simulink model "playback_data"  (R2015a)
settings: Solver=FixedStepDiscrete  SolverMode=SingleTasking  StartTime=76  StopTime=110  FixedStep=sample_time  RelTol=1e-3
undefined symbols (not defined in the file): A1_notch_f1, A2_notch_f1, A_kalman_swing_load, A_kalman_transverse, A_kalman_vertical, A_lpf_accelerometer, A_lpf_dtau, A_lpf_fourbar_angles, A_lpf_imu, A_lpf_lateral_angle, B1_lpf_accelerometer, B1_lpf_dtau, B1_lpf_fourbar_angles, B1_lpf_imu, B1_lpf_lateral_angle, B1_notch_f1, B2_lpf_accelerometer, B2_lpf_dtau, B2_lpf_fourbar_angles, B2_lpf_imu, B2_lpf_lateral_angle, B2_notch_f1, B_dx_versus_x0, B_kalman_swing_load, B_kalman_transverse, B_kalman_vertical, backwards_K_sag_of_t, backwards_P_sag_of_t, C_kalman_swing_load, C_kalman_transverse, C_kalman_vertical, com_leg_motor, com_torso, contact_threshold, control_start_time, d_ankle_to_foot, d_vertical_com, desired_com_forward_velocity, desired_com_lateral_velocity, desired_initial_leg_roll_left, desired_initial_leg_roll_right, desired_stance_beta2, desired_standing_torso_pitch, desired_standing_torso_roll, desired_standing_z, desired_torso_pitch, desired_torso_roll, Discrete, enable_bouncing, fcut_contact, fdesignblkfcn, forward_dx_of_dxstar, forward_x_of_dxstar, g, gcbh, HIP_MTR_MAX_CONT_TORQUE, HIP_MTR_MAX_TORQUE, i_leg_motor, i_robot, i_torso ... (+78)
libraries: simulink x65, dsparch4 x18, ctrlSharedLib x14, dspfdesign x4
(part 4 of 13)

== system playback_data/Control1/Filter Velocities ==
  raw dq : Inport
  Demux : Demux  Outputs=3
  Demux1 : Demux  Outputs=3
  Demux2 : Demux  Outputs=2
  Demux3 : Demux  Outputs=2
  Fourbar : Selector  InputPortWidth=13  Indices=[1 2 3 4 5 6 7 8]
  Fourbar Velocity Filter : Scope  NumInputPorts=4
      settings: YMin=-0.55~-0.4~-0.4~-0.6  YMax=0.25~0.7~0.45~0.5  SaveName=ScopeData14  SampleInput=on
  IMU Two Pole Filter : DiscreteTransferFcn  Numerator=[A_lpf_imu 0 0]  Denominator=[1 B1_lpf_imu B2_lpf_imu]  SampleTime=sample_time
  Lateral : Selector  InputPortWidth=13  Indices=[9 10]
  Lateral Angle Two Pole Filter1 : DiscreteTransferFcn  Numerator=[A_lpf_lateral_angle 0 0]  Denominator=[1 B1_lpf_lateral_angle B2_lpf_lateral_angle]  SampleTime=sample_time
  Lateral Angle Two Pole Filter2 : DiscreteTransferFcn  Numerator=[A_lpf_fourbar_angles 0 0]  Denominator=[1 B1_lpf_fourbar_angles B2_lpf_fourbar_angles]  SampleTime=sample_time
  Leg Roll Velocity Filter : Scope  NumInputPorts=2
      settings: YMin=-0.225~-1.5  YMax=0.175~2.25  SaveName=LegRollFilter  SampleInput=on
  Mux : Mux  Inputs=3
  Mux{25..33} (9 alike) : Mux  Inputs=2
  Selector1 : Selector  InputPortWidth=8  Indices=[1 2]
  Selector2 : Selector  InputPortWidth=8  Indices=[3 4]
  Selector3 : Selector  InputPortWidth=8  Indices=[5 6]
  Selector34 : Selector  InputPortWidth=8  Indices=[1 2]
  Selector35 : Selector  InputPortWidth=8  Indices=[3 4]
  Selector36 : Selector  InputPortWidth=8  Indices=[5 6]
  Selector37 : Selector  InputPortWidth=8  Indices=[7 8]
  Selector4 : Selector  InputPortWidth=8  Indices=[7 8]
  Torso Orientation : Selector  InputPortWidth=13  Indices=[11 12 13]
  Torso Orientation Filter : Scope  NumInputPorts=3
      settings: YMin=-0.2~-0.03~-0.15  YMax=0.125~0.0275~0.15  SaveName=ScopeData13  SampleInput=on
  filtered dq : Outport
  wires:
  Lateral Angle Two Pole Filter2/1 -> Selector4/1, Selector3/1, Selector2/1, Selector1/1, Mux/1
  IMU Two Pole Filter/1 -> Demux1/1, Mux/3
  Mux/1 -> filtered dq/1
  raw dq/1 -> Fourbar/1, Torso Orientation/1, Lateral/1
  Lateral/1 -> Demux2/1, Lateral Angle Two Pole Filter1/1
  Torso Orientation/1 -> IMU Two Pole Filter/1, Demux/1
  Lateral Angle Two Pole Filter1/1 -> Demux3/1, Mux/2
  Mux25/1 -> Torso Orientation Filter/1
  Mux27/1 -> Torso Orientation Filter/3
  Mux26/1 -> Torso Orientation Filter/2
  Mux30/1 -> Fourbar Velocity Filter/1
  Mux32/1 -> Fourbar Velocity Filter/3
  Mux31/1 -> Fourbar Velocity Filter/2
  Mux33/1 -> Fourbar Velocity Filter/4
  Selector34/1 -> Mux30/1
  Fourbar/1 -> Selector34/1, Selector35/1, Selector36/1, Selector37/1, Lateral Angle Two Pole Filter2/1
  Selector35/1 -> Mux31/1
  Selector36/1 -> Mux32/1
  Selector37/1 -> Mux33/1
  Mux28/1 -> Leg Roll Velocity Filter/1
  Mux29/1 -> Leg Roll Velocity Filter/2
  Demux/1 -> Mux25/1
  Demux/2 -> Mux26/1
  Demux/3 -> Mux27/1
  Demux1/1 -> Mux25/2
  Demux1/2 -> Mux26/2
  Demux1/3 -> Mux27/2
  Demux2/2 -> Mux29/1
  Demux2/1 -> Mux28/1
  Demux3/1 -> Mux28/2
  Demux3/2 -> Mux29/2
  Selector4/1 -> Mux33/2
  Selector3/1 -> Mux32/2
  Selector2/1 -> Mux31/2
  Selector1/1 -> Mux30/2

== system playback_data/Control/Actuator Control with Torque SEA commands/Compare SEA Signals ==
  Desired : Inport
  Measured : Inport  Port=2
  Demux : Demux
  Demux1 : Demux
  Mux{6..9} (4 alike) : Mux  Inputs=2
  RB : Outport
  RF : Outport  Port=2
  LB : Outport  Port=3
  LF : Outport  Port=4
  wires:
  Demux/3 -> Mux8/1
  Demux/2 -> Mux7/1
  Demux1/1 -> Mux6/2
  Demux/1 -> Mux6/1
  Demux/4 -> Mux9/1
  Demux1/4 -> Mux9/2
  Measured/1 -> Demux1/1
  Demux1/2 -> Mux7/2
  Desired/1 -> Demux/1
  Demux1/3 -> Mux8/2
  Mux6/1 -> RB/1
  Mux7/1 -> RF/1
  Mux9/1 -> LF/1
  Mux8/1 -> LB/1

== system playback_data/Control/Actuator Control with Torque SEA commands/Compare Signals ==
  Measurement : Inport
  Filtered : Inport  Port=2
  Expected : Inport  Port=3
  Demux : Demux
  Demux1 : Demux
  Demux2 : Demux
  Mux{6..9} (4 alike) : Mux  Inputs=3
  RB : Outport
  RF : Outport  Port=2
  LB : Outport  Port=3
  LF : Outport  Port=4
  wires:
  Mux8/1 -> LB/1
  Mux9/1 -> LF/1
  Mux7/1 -> RF/1
  Mux6/1 -> RB/1
  Demux1/3 -> Mux8/2
  Measurement/1 -> Demux/1
  Demux1/2 -> Mux7/2
  Filtered/1 -> Demux1/1
  Demux1/4 -> Mux9/2
  Demux/4 -> Mux9/1
  Demux/1 -> Mux6/1
  Demux1/1 -> Mux6/2
  Demux/2 -> Mux7/1
  Demux/3 -> Mux8/1
  Expected/1 -> Demux2/1
  Demux2/1 -> Mux6/3
  Demux2/2 -> Mux7/3
  Demux2/3 -> Mux8/3
  Demux2/4 -> Mux9/3

== system playback_data/Control/Actuator Control with Torque SEA commands/Compare Torque Derivative Signals ==
  Measured : Inport
  Filtered : Inport  Port=2
  Expected : Inport  Port=3
  Demux : Demux
  Demux1 : Demux
  Demux2 : Demux
  Mux{6..9} (4 alike) : Mux  Inputs=3
  RB : Outport
  RF : Outport  Port=2
  LB : Outport  Port=3
  LF : Outport  Port=4
  wires:
  Demux2/4 -> Mux9/3
  Demux2/3 -> Mux8/3
  Demux2/2 -> Mux7/3
  Demux2/1 -> Mux6/3
  Expected/1 -> Demux2/1
  Demux/3 -> Mux8/1
  Demux/2 -> Mux7/1
  Demux1/1 -> Mux6/2
  Demux/1 -> Mux6/1
  Demux/4 -> Mux9/1
  Demux1/4 -> Mux9/2
  Filtered/1 -> Demux1/1
  Demux1/2 -> Mux7/2
  Measured/1 -> Demux/1
  Demux1/3 -> Mux8/2
  Mux6/1 -> RB/1
  Mux7/1 -> RF/1
  Mux9/1 -> LF/1
  Mux8/1 -> LB/1

== system playback_data/Control/Actuator Control with Torque SEA commands/Compare Velocities ==
  Desired : Inport
  Measured : Inport  Port=2
  Demux : Demux
  Demux1 : Demux
  Mux{6..9} (4 alike) : Mux  Inputs=2
  RB : Outport
  RF : Outport  Port=2
  LB : Outport  Port=3
  LF : Outport  Port=4
  wires:
  Demux1/3 -> Mux8/2
  Desired/1 -> Demux/1
  Demux1/2 -> Mux7/2
  Measured/1 -> Demux1/1
  Demux1/4 -> Mux9/2
  Demux/4 -> Mux9/1
  Demux/1 -> Mux6/1
  Demux1/1 -> Mux6/2
  Demux/2 -> Mux7/1
  Demux/3 -> Mux8/1
  Mux6/1 -> RB/1
  Mux7/1 -> RF/1
  Mux8/1 -> LB/1
  Mux9/1 -> LF/1

== system playback_data/Control/Actuator Control with Torque SEA commands/Contact Velocities ==
  Contact [1/0] x4 : Inport
  Velocities [rad/s] x4 : Inport  Port=2
  Demux : Demux
  Demux1 : Demux
  Mux : Mux
  Velocity on Contact : Subsystem
  Velocity on Contact1 : Subsystem
  Velocity on Contact2 : Subsystem
  Velocity on Contact3 : Subsystem
  Contact Velocities [rad/s] x4 : Outport
  wires:
  Mux/1 -> Contact Velocities [rad/s] x4/1
  Demux/2 -> Velocity on Contact1/Trigger
  Velocity on Contact/1(out) -> Mux/1
  Contact [1/0] x4/1 -> Demux/1
  Velocity on Contact1/1(out) -> Mux/2
  Demux/3 -> Velocity on Contact2/Trigger
  Demux/4 -> Velocity on Contact3/Trigger
  Demux/1 -> Velocity on Contact/Trigger
  Velocity on Contact3/1(out) -> Mux/4
  Velocity on Contact2/1(out) -> Mux/3
  Velocities [rad/s] x4/1 -> Demux1/1
  Demux1/1 -> Velocity on Contact/1(in)
  Demux1/2 -> Velocity on Contact1/1(in)
  Demux1/3 -> Velocity on Contact2/1(in)
  Demux1/4 -> Velocity on Contact3/1(in)

== system playback_data/Control/Actuator Control with Torque SEA commands/Desired Torque Derivative ==
  Signal x4 : Inport
  Reset [1/0] x4 : Inport  Port=2
  Demux : Demux
  Demux1 : Demux
  Gain1 : Gain  Gain=1/sample_time
  Logical Operator : Logic  Operator=NOT  AllPortsSameDT=off  OutDataTypeStr=boolean
  Mux : Mux
  Product : Product
  difference : simulink/Discrete/Difference  ICPrevInput=0.0  InputProcessing=Inherited  OutMin=[]  OutMax=[]  OutDataType=fixdt(1, 16)  OutScaling=2^-10  DoSatur=off
  two_pole_filter{,1..3} (4 alike) : DiscreteTransferFcn  Numerator=[A_lpf_dtau 0 0]  Denominator=[1 B1_lpf_dtau B2_lpf_dtau]  ExternalReset=Rising  SampleTime=sample_time
      settings: InputPortMap=u0,r7
  Derivative x4 : Outport
  wires:
  Demux/1 -> two_pole_filter/1
  difference/1 -> Product/1
  Mux/1 -> Derivative x4/1
  Signal x4/1 -> Gain1/1
  Gain1/1 -> difference/1
  Logical Operator/1 -> Product/2
  Reset [1/0] x4/1 -> Demux1/1, Logical Operator/1
  two_pole_filter/1 -> Mux/1
  Product/1 -> Demux/1
  two_pole_filter1/1 -> Mux/2
  two_pole_filter2/1 -> Mux/3
  two_pole_filter3/1 -> Mux/4
  Demux/2 -> two_pole_filter1/1
  Demux/3 -> two_pole_filter2/1
  Demux/4 -> two_pole_filter3/1
  Demux1/1 -> two_pole_filter/2
  Demux1/2 -> two_pole_filter1/2
  Demux1/3 -> two_pole_filter2/2
  Demux1/4 -> two_pole_filter3/2

== system playback_data/Control/Actuator Control with Torque SEA commands/Expected Forces on Foot ==
  R/L Leg Length [m] x2 : Inport
  R/L Leg Width [m] x2 : Inport  Port=2
  Torques on Load [Nm] x4 : Inport  Port=3
  Divide : Product  Inputs=/*
  Divide1 : Product  Inputs=/*
  Gain3 : Gain  Gain=-1
  Gain6 : Gain  Gain=-1
  Selector2 : Selector  InputPortWidth=4  Indices=[1 3]
  Selector7 : Selector  InputPortWidth=4  Indices=[2 4]
  Sum5 : Sum  Inputs=|-+
  Sum6 : Sum  Inputs=++|
  R/L Orthogonal Force [N] x2 : Outport
  R/L Axial Force [N] x2 : Outport  Port=2
  wires:
  Gain6/1 -> R/L Orthogonal Force [N] x2/1
  Gain3/1 -> R/L Axial Force [N] x2/1
  Sum5/1 -> Divide1/2
  Selector7/1 -> Sum6/2, Sum5/2
  Sum6/1 -> Divide/2
  Selector2/1 -> Sum5/1, Sum6/1
  Divide1/1 -> Gain3/1
  Torques on Load [Nm] x4/1 -> Selector2/1, Selector7/1
  R/L Leg Width [m] x2/1 -> Divide1/1
  R/L Leg Length [m] x2/1 -> Divide/1
  Divide/1 -> Gain6/1

== system playback_data/Control/Actuator Control with Torque SEA commands/Load Torque Kalman Filter ==
  Measured Spring Torque [Nm] x4 : Inport
  Load Position [rad/s] x4 : Inport  Port=2
  Load Velocity [rad/s] x4 : Inport  Port=3
  Reset [1/0] x4 : Inport  Port=4
  Constant{,1..3} (4 alike) : Constant  Value=P0_kalman_swing_load
  Demux2 : Demux
  Difference{,1..3} (4 alike) : simulink/Discrete/Difference  ICPrevInput=0.0  InputProcessing=Inherited  OutMin=[]  OutMax=[]  OutDataType=fixdt(1, 16)  OutScaling=2^-10  DoSatur=off
  Gain{1..4} (4 alike) : Gain  Gain=1/mean(j_segments)
  Gain5 : Gain  Gain=mean(j_segments)
  MATLAB Function : MATLAB Function  TreatAsAtomicUnit=on
  Mux : Mux
  Mux{1,3,5,7} (4 alike) : Mux  Inputs=2
  Mux{2,4,6,8} (4 alike) : Mux  Inputs=3
  Selector : Selector  InputPortWidth=4  Indices=[1]
  Selector{1..3,12} (4 alike) : Selector  InputPortWidth=3  Indices=[3]
  Selector10 : Selector  InputPortWidth=4  Indices=[2]
  Selector11 : Selector  InputPortWidth=4  Indices=[3]
  Selector13 : Selector  InputPortWidth=4  Indices=[3]
  Selector14 : Selector  InputPortWidth=4  Indices=[4]
  Selector15 : Selector  InputPortWidth=4  Indices=[4]
  Selector4 : Selector  InputPortWidth=4  Indices=[1]
  Selector5 : Selector  InputPortWidth=4  Indices=[1]
  Selector6 : Selector  InputPortWidth=4  Indices=[2]
  Selector7 : Selector  InputPortWidth=4  Indices=[3]
  Selector8 : Selector  InputPortWidth=4  Indices=[4]
  Selector9 : Selector  InputPortWidth=4  Indices=[2]
  Swing Load Kalman Filter{,1..3} (4 alike) : ctrlSharedLib/Kalman Filter  TimeDomain=Discrete-Time  UseCurrentEstimator=on  ModelSource=Individual A, B, C, D matrices  ModelSourceVariable=A_kf  A=A_kalman_swing_load  B=B_kalman_swing_load  C=C_kalman_swing_load  D=0  NumberOfStates=2  NumberOfInputs=1  NumberOfOutputs=2  InitialEstimateSource=Input port  X0=initial_dx_estimate  P0=P0_kalman_transverse  UseK=off  UseGH=on  NumberOfProcessNoiseInputs=1  G=G_kalman_swing_load  TimeInvariantG=on  H=0  TimeInvariantH=on  Q=Q_kalman_SEA_torque_difference  TimeInvariantQ=on  R=1  TimeInvariantR=off  N=0  TimeInvariantN=on  AddInputPort=on  AddEnablePort=off  ExternalReset=Rising  OutputEstimatedY=off  OutputP=off  Ts=sample_time
  Load Torques [Nm] x4 : Outport
  wires:
  Mux6/1 -> Swing Load Kalman Filter/3
  Mux5/1 -> Swing Load Kalman Filter/2
  Difference/1 -> Swing Load Kalman Filter/1
  Demux2/1 -> Gain3/1, Mux5/2, Difference/1
  Swing Load Kalman Filter/1 -> Selector12/1
  Selector12/1 -> Mux/1
  Mux2/1 -> Swing Load Kalman Filter1/3
  Mux1/1 -> Swing Load Kalman Filter1/2
  Difference1/1 -> Swing Load Kalman Filter1/1
  Demux2/2 -> Gain1/1, Mux1/2, Difference1/1
  Gain1/1 -> Mux2/3
  Mux4/1 -> Swing Load Kalman Filter2/3
  Mux3/1 -> Swing Load Kalman Filter2/2
  Difference2/1 -> Swing Load Kalman Filter2/1
  Demux2/3 -> Difference2/1, Mux3/2, Gain2/1
  Gain2/1 -> Mux4/3
  Mux8/1 -> Swing Load Kalman Filter3/3
  Mux7/1 -> Swing Load Kalman Filter3/2
  Difference3/1 -> Swing Load Kalman Filter3/1
  Demux2/4 -> Difference3/1, Mux7/2, Gain4/1
  Gain4/1 -> Mux8/3
  Swing Load Kalman Filter1/1 -> Selector1/1
  Swing Load Kalman Filter3/1 -> Selector3/1
  Swing Load Kalman Filter2/1 -> Selector2/1
  Mux/1 -> Gain5/1
  Selector1/1 -> Mux/2
  Selector2/1 -> Mux/3
  Selector3/1 -> Mux/4
  Reset [1/0] x4/1 -> [Reset]
  Load Velocity [rad/s] x4/1 -> [LoadVelocities]
  Measured Spring Torque [Nm] x4/1 -> MATLAB Function/1(spring_torques), Demux2/1
  Gain5/1 -> Load Torques [Nm] x4/1
  Gain3/1 -> Mux6/3
  Load Position [rad/s] x4/1 -> [LoadPositions]
  [LoadPositions] -> Selector/1
  [LoadVelocities] -> Selector4/1
  Selector/1 -> Mux6/1, Mux5/1
  Selector4/1 -> Mux6/2
  [Reset] -> Selector5/1
  Selector5/1 -> Swing Load Kalman Filter/5
  [Reset] -> Selector6/1
  Selector6/1 -> Swing Load Kalman Filter1/5
  [Reset] -> Selector7/1
  Selector7/1 -> Swing Load Kalman Filter2/5
  [Reset] -> Selector8/1
  Selector8/1 -> Swing Load Kalman Filter3/5
  [LoadVelocities] -> Selector9/1
  [LoadPositions] -> Selector10/1
  [LoadVelocities] -> Selector11/1
  [LoadPositions] -> Selector13/1
  [LoadVelocities] -> Selector14/1
  [LoadPositions] -> Selector15/1
  Selector15/1 -> Mux8/1, Mux7/1
  Selector13/1 -> Mux4/1, Mux3/1
  Selector11/1 -> Mux4/2
  Selector14/1 -> Mux8/2
  Selector9/1 -> Mux2/2
  Selector10/1 -> Mux2/1, Mux1/1
  Constant/1 -> Swing Load Kalman Filter1/4
  MATLAB Function/1(R1) -> [R1]
  MATLAB Function/2(R2) -> [R2]
  MATLAB Function/3(R3) -> [R3]
  MATLAB Function/4(R4) -> [R4]
  [R2] -> Swing Load Kalman Filter1/6
  [R1] -> Swing Load Kalman Filter/6
  Constant1/1 -> Swing Load Kalman Filter/4
  [R3] -> Swing Load Kalman Filter2/6
  Constant2/1 -> Swing Load Kalman Filter2/4
  Constant3/1 -> Swing Load Kalman Filter3/4
  [R4] -> Swing Load Kalman Filter3/6

== system playback_data/Control/Actuator Control with Torque SEA commands/Lowpass Filter ==
  In : Inport
  Generated Filter Block : dsparch4/Biquad Filter  Tag=BlockMethodSubSystem  IIRFiltStruct=Direct form II  CoeffSource=Specify via dialog  BiQuadCoeffs=[1.0054190789171848 -2 1.0054190789171853 1 -1.9557970115108714 0.95685429506963915]  a0Flag=Warning  IC=0  ICnum=0  ICden=0  denAccumFracLength=30  denProdOutputFracLength=30  secondMemoryFracLength=15  roundingMode=Floor  overflowMode=off  ScaleValues=[0.0010519560093213882;92.733879468734756]  optimizeScaleValues=off  ScaleValueMode=Specify via input port (g)  scaleValueFracLength=14  FilterSource=Specify via dialog  FilterObject=Hm_biquad
  Out : Outport
  wires:
  Generated Filter Block/1 -> Out/1
  In/1 -> Generated Filter Block/1

== system playback_data/Control/Actuator Control with Torque SEA commands/Lowpass Filter1 ==
  In : Inport
  Generated Filter Block : dsparch4/Biquad Filter  Tag=BlockMethodSubSystem  IIRFiltStruct=Direct form II  CoeffSource=Specify via dialog  BiQuadCoeffs=[1.0054190789171848 -2 1.0054190789171853 1 -1.9557970115108714 0.95685429506963915]  a0Flag=Warning  IC=0  ICnum=0  ICden=0  denAccumFracLength=30  denProdOutputFracLength=30  secondMemoryFracLength=15  roundingMode=Floor  overflowMode=off  ScaleValues=[0.0010519560093213882;92.733879468734756]  optimizeScaleValues=off  ScaleValueMode=Specify via input port (g)  scaleValueFracLength=14  FilterSource=Specify via dialog  FilterObject=Hm_biquad
  Out : Outport
  wires:
  In/1 -> Generated Filter Block/1
  Generated Filter Block/1 -> Out/1

== system playback_data/Control/Actuator Control with Torque SEA commands/Lowpass Filter2 ==
  In : Inport
  Generated Filter Block : dsparch4/Biquad Filter  Tag=BlockMethodSubSystem  IIRFiltStruct=Direct form II  CoeffSource=Specify via dialog  BiQuadCoeffs=[0.42638734887522584 0.71004939850960869 0.42638734887522595 1 0.054295561672899631 0.19751119790393634]  a0Flag=Warning  IC=0  ICnum=0  ICden=0  denAccumFracLength=30  denProdOutputFracLength=30  secondMemoryFracLength=15  roundingMode=Floor  overflowMode=off  ScaleValues=[0.80099018345858064;1]  optimizeScaleValues=off  ScaleValueMode=Specify via input port (g)  scaleValueFracLength=14  FilterSource=Specify via dialog  FilterObject=Hm_biquad
  Out : Outport
  wires:
  In/1 -> Generated Filter Block/1
  Generated Filter Block/1 -> Out/1

== system playback_data/Control/Actuator Control with Torque SEA commands/Lowpass Filter5 ==
  In : Inport
  Generated Filter Block : dsparch4/Biquad Filter  Tag=BlockMethodSubSystem  IIRFiltStruct=Direct form II  CoeffSource=Specify via dialog  BiQuadCoeffs=[1.0054190789171848 -2 1.0054190789171853 1 -1.9557970115108714 0.95685429506963915]  a0Flag=Warning  IC=0  ICnum=0  ICden=0  denAccumFracLength=30  denProdOutputFracLength=30  secondMemoryFracLength=15  roundingMode=Floor  overflowMode=off  ScaleValues=[0.0010519560093213882;92.733879468734756]  optimizeScaleValues=off  ScaleValueMode=Specify via input port (g)  scaleValueFracLength=14  FilterSource=Specify via dialog  FilterObject=Hm_biquad
  Out : Outport
  wires:
  In/1 -> Generated Filter Block/1
  Generated Filter Block/1 -> Out/1

== system playback_data/Control/Actuator Control with Torque SEA commands/Lowpass Filter6 ==
  In : Inport
  Generated Filter Block : dsparch4/Biquad Filter  Tag=BlockMethodSubSystem  IIRFiltStruct=Direct form II  CoeffSource=Specify via dialog  BiQuadCoeffs=[1.0054190789171848 -2 1.0054190789171853 1 -1.9557970115108714 0.95685429506963915]  a0Flag=Warning  IC=0  ICnum=0  ICden=0  denAccumFracLength=30  denProdOutputFracLength=30  secondMemoryFracLength=15  roundingMode=Floor  overflowMode=off  ScaleValues=[0.0010519560093213882;92.733879468734756]  optimizeScaleValues=off  ScaleValueMode=Specify via input port (g)  scaleValueFracLength=14  FilterSource=Specify via dialog  FilterObject=Hm_biquad
  Out : Outport
  wires:
  Generated Filter Block/1 -> Out/1
  In/1 -> Generated Filter Block/1

== system playback_data/Control/Actuator Control with Torque SEA commands/Measured Forces on Foot ==
  R/L Leg Length [m] x2 : Inport
  R/L Leg Width [m] x2 : Inport  Port=2
  Torques on Load [Nm] x4 : Inport  Port=3
  Divide : Product  Inputs=/*
  Divide1 : Product  Inputs=/*
  Gain3 : Gain  Gain=-1
  Gain6 : Gain  Gain=-1
  Selector2 : Selector  InputPortWidth=4  Indices=[1 3]
  Selector7 : Selector  InputPortWidth=4  Indices=[2 4]
  Sum5 : Sum  Inputs=|-+
  Sum6 : Sum  Inputs=++|
  R/L Orthogonal Force [N] x2 : Outport
  R/L Axial Force [N] x2 : Outport  Port=2
  wires:
  Divide/1 -> Gain6/1
  R/L Leg Length [m] x2/1 -> Divide/1
  R/L Leg Width [m] x2/1 -> Divide1/1
  Torques on Load [Nm] x4/1 -> Selector7/1, Selector2/1
  Divide1/1 -> Gain3/1
  Selector2/1 -> Sum6/1, Sum5/1
  Sum6/1 -> Divide/2
  Selector7/1 -> Sum5/2, Sum6/2
  Sum5/1 -> Divide1/2
  Gain3/1 -> R/L Axial Force [N] x2/1
  Gain6/1 -> R/L Orthogonal Force [N] x2/1

== system playback_data/Control/Actuator Control with Torque SEA commands/SEA Controller (Torque) ==
  phi_load [rad] x4 : Inport
  phi_gear [rad] x4 : Inport  Port=2
  dphi_load [rad/s] x4 : Inport  Port=3
  dphi_gear [rad/s] x4 : Inport  Port=4
  tau_des sagittal [Nm] x4 : Inport  Port=5
  dtau_des sagittal [Nm] x4 : Inport  Port=6
  Abs : Abs
  Antiresonance Compensation : Subsystem
  Friction Compensation : Subsystem
  Loaded Unloaded Switch : Subsystem
  P gain ramp : Lookup_n-D  NumberOfTableDimensions=1  BreakpointsForDimension1=[0,65,350,700]  Table=0.60*[0.3, 0.3, 6.0, 6.0]  InternalRulePriority=Speed  RndMeth=Simplest  InputSameDT=on
  Product : Product  SampleTime=sample_time  RndMeth=Zero
  Product2 : Product  RndMeth=Zero
  Spring Stiffness : Gain  Gain=k_sea_low
  Spring Stiffness 1 : Gain  Gain=k_sea_low
  Sum1 : Sum  Inputs=-+|
  Sum10 : Sum  Inputs=|++
  Sum2 : Sum  Inputs=|+-
  Sum3 : Sum  Inputs=++|
  Sum5 : Sum  Inputs=|+-
  Sum6 : Sum  Inputs=-+|
  Sum7 : Sum  Inputs=+|+
  Torque Limiter (outside) 1 : Saturate  UpperLimit=max_sagittal_loaded_torque  LowerLimit=-max_sagittal_loaded_torque
      settings: AttributesFormatString=Hi: %<UpperLimit>\nLo: %<LowerLimit>
  Torque Limiter (outside) 3 : Saturate  UpperLimit=max_sagittal_unloaded_torque  LowerLimit=-max_sagittal_unloaded_torque
      settings: AttributesFormatString=Hi: %<UpperLimit>\nLo: %<LowerLimit>
  Torque Threshold : simulink/Logic and Bit Operations/Compare To Constant  relop=>=  const=loaded_unloaded_torque_threshold  OutDataTypeStr=boolean
  critical damping : Subsystem
  tau_cmd sagittal [Nm] x4 : Outport
  tau_measured [Nm] x4 : Outport  Port=2
  wires:
  Product2/1 -> Sum7/2
  Sum2/1 -> Product2/2
  Sum5/1 -> Product/2
  dphi_gear [rad/s] x4/1 -> Friction Compensation/1(Motor Velocity [rad/s]), Sum6/2
  dphi_load [rad/s] x4/1 -> Sum6/1
  Spring Stiffness 1/1 -> Sum2/2
  Sum6/1 -> Spring Stiffness 1/1
  dtau_des sagittal [Nm] x4/1 -> Sum2/1
  tau_des sagittal [Nm] x4/1 -> Sum5/1
  phi_gear [rad] x4/1 -> Sum1/2
  phi_load [rad] x4/1 -> Sum1/1
  Sum1/1 -> Spring Stiffness/1
  Spring Stiffness/1 -> Sum3/1, Sum5/2, Abs/1, tau_measured [Nm] x4/1
  Sum10/1 -> Antiresonance Compensation/1(Torque), Torque Limiter (outside) 1/1
  P gain ramp/1 -> critical damping/1(p gain), Product/1
  Product/1 -> Sum7/1
  Sum7/1 -> Sum3/2
  Torque Limiter (outside) 1/1 -> Loaded Unloaded Switch/1(Loaded Signal)
  Torque Limiter (outside) 3/1 -> Loaded Unloaded Switch/2(Unloaded Signal)
  Antiresonance Compensation/1(Filtered Torque) -> Torque Limiter (outside) 3/1
  Friction Compensation/1(Friction Compensation [Nm]) -> Sum10/2
  Loaded Unloaded Switch/1(Signal) -> tau_cmd sagittal [Nm] x4/1
  Torque Threshold/1 -> Loaded Unloaded Switch/3(Loaded/Unloaded [1/0] x4)
  Abs/1 -> P gain ramp/1, Torque Threshold/1
  Sum3/1 -> Sum10/1
  critical damping/1(d gain) -> Product2/1

== system playback_data/Control/Actuator Control with Torque SEA commands/SEA Controller (Velocity) ==
  phi_load [rad] x4 : Inport
  phi_gear [rad] x4 : Inport  Port=2
  dphi_load [rad/s] x4 : Inport  Port=3
  tau_des sagittal [Nm] x4 : Inport  Port=4
  dtau_des sagittal [Nm] x4 : Inport  Port=5
  Reset SEA Control [1/0] x4 : Inport  Port=6
  Stance (1) or Swing (0) x4 : Inport  Port=7
  Demux : Demux
  Demux1 : Demux
  Demux2 : Demux
  Feedback : Scope  NumInputPorts=4
      settings: YMin=-4~-0.9~-5~-5  YMax=4.5~1~5~5  SaveName=ScopeData7  SampleInput=on
  Feedforward : Scope  NumInputPorts=4
      settings: YMin=-4~-0.9~-5~-5  YMax=4.5~1~5~5  SaveName=ScopeData4  SampleInput=on
  Gain3 : Gain  Gain=1./k_sea_low
  Integrator : Subsystem
  Kp : Constant  Value=0.016
  Lowpass Filter (Stance) : Subsystem  DialogController=fdesignblkfcn  InitFcn=fdesignblkfcn(gcbh, {'InitFcn'});  mask(Lowpass Filter){}
      mask help: Design a lowpass filter
      settings: CopyFcn=fdesignblkfcn(gcbh, {'CopyFcn'});
      mask Help: helpview(mapfilelocation('dsp'), 'dsplowpassfilter');
      mask Display: disp('Lowpass')
  Lowpass Filter (Swing) : Subsystem  DialogController=fdesignblkfcn  InitFcn=fdesignblkfcn(gcbh, {'InitFcn'});  mask(Lowpass Filter){}
      mask help: Design a lowpass filter
      settings: CopyFcn=fdesignblkfcn(gcbh, {'CopyFcn'});
      mask Help: helpview(mapfilelocation('dsp'), 'dsplowpassfilter');
      mask Display: disp('Lowpass')
  Nonlinear Spring Force : MATLAB Function  TreatAsAtomicUnit=on
  Product : Product
  Stance Swing : Scope  NumInputPorts=4
      settings: YMin=-4~-0.9~-5~-5  YMax=4.5~1~5~5  SaveName=ScopeData5  SampleInput=on
  Stance or Swing : Subsystem
  Stance or Swing1 : Subsystem
  Stance or Swing2 : Subsystem
  Sum1 : Sum  Inputs=-+|
  Sum10 : Sum  Inputs=++|
  Sum4 : Sum  Inputs=|++
  Sum5 : Sum  Inputs=|+-
  Sum6 : Sum  Inputs=|++
  Ti : Gain  Gain=1/0.150
  Torque Limiter (stance) : Saturate  UpperLimit=700  LowerLimit=-700
      settings: AttributesFormatString=Hi: %<UpperLimit>\nLo: %<LowerLimit>
  Torque Limiter (swing) : Saturate  UpperLimit=80  LowerLimit=-80
      settings: AttributesFormatString=Hi: %<UpperLimit>\nLo: %<LowerLimit>
  Velocity Notch Filter (Swing) : dspfdesign/Notch-Peak Filter  Specification=Quality factor and center frequency  Bandwidth=27  QualityFactor=2.5  CenterFrequency=27  BandwidthCoefficient=0.72654  CenterFrequencyCoefficient=0  Output=Notch  InheritSampleRate=off  SampleRate=update_freq  SimulateUsing=Code generation
  Velocity Command [rad/s] x4 : Outport  PortDimensions=4
  tau_measured [Nm] x4 : Outport  Port=2
  wires:
  Sum1/1 -> Nonlinear Spring Force/1(deflections)
  Nonlinear Spring Force/1(tau_sea) -> tau_measured [Nm] x4/1, Sum5/2
  Product/1 -> Ti/1, Sum10/1
  Sum6/1 -> Stance or Swing1/2(Signal True x4), Velocity Notch Filter (Swing)/1
  Gain3/1 -> Sum4/1
  dtau_des sagittal [Nm] x4/1 -> Gain3/1
  Reset SEA Control [1/0] x4/1 -> Integrator/2(Reset [1/0])
  Sum5/1 -> Product/1
  Integrator/1(Integrated) -> Sum10/2
  Ti/1 -> Integrator/1(Signal)
  dphi_load [rad/s] x4/1 -> Sum4/2
  Sum4/1 -> Lowpass Filter (Stance)/1(In), Lowpass Filter (Swing)/1(In)
  Lowpass Filter (Stance)/1(Out) -> Stance or Swing2/2(Signal True x4), Demux1/1
  Kp/1 -> Product/2
  Stance or Swing/1(Selected x4) -> Sum5/1
  Torque Limiter (swing)/1 -> Stance or Swing/3(Signal False x4)
  Torque Limiter (stance)/1 -> Stance or Swing/2(Signal True x4)
  Stance or Swing1/1(Selected x4) -> Velocity Command [rad/s] x4/1
  Velocity Notch Filter (Swing)/1 -> Stance or Swing1/3(Signal False x4)
  Demux/4 -> Feedback/4
  Demux/3 -> Feedback/3
  Demux/2 -> Feedback/2
  Demux/1 -> Feedback/1
  Demux1/1 -> Feedforward/1
  Demux1/2 -> Feedforward/2
  Demux1/3 -> Feedforward/3
  Demux1/4 -> Feedforward/4
  tau_des sagittal [Nm] x4/1 -> Torque Limiter (stance)/1, Torque Limiter (swing)/1
  phi_gear [rad] x4/1 -> Sum1/2
  phi_load [rad] x4/1 -> Sum1/1
  Stance (1) or Swing (0) x4/1 -> Demux2/1, Stance or Swing2/1(True/False x4), Stance or Swing1/1(True/False x4), Stance or Swing/1(True/False x4)
  Demux2/3 -> Stance Swing/3
  Demux2/2 -> Stance Swing/2
  Demux2/1 -> Stance Swing/1
  Demux2/4 -> Stance Swing/4
  Sum10/1 -> Demux/1, Sum6/1
  Lowpass Filter (Swing)/1(Out) -> Stance or Swing2/3(Signal False x4)
  Stance or Swing2/1(Selected x4) -> Sum6/2

== system playback_data/Control/Actuator Control with Torque SEA commands/Stance or Swing1 ==
  True/False x4 : Inport
  Signal True x4 : Inport  Port=2
  Signal False x4 : Inport  Port=3
  Demux : Demux
  Demux1 : Demux
  Demux2 : Demux
  Mux : Mux
  Switch{,1..3} (4 alike) : Switch  Criteria=u2 ~= 0
  Selected x4 : Outport
  wires:
  Switch3/1 -> Mux/4
  Switch2/1 -> Mux/3
  Switch1/1 -> Mux/2
  Switch/1 -> Mux/1
  Demux1/4 -> Switch3/2
  Demux1/3 -> Switch2/2
  Demux1/2 -> Switch1/2
  Demux1/1 -> Switch/2
  Demux2/4 -> Switch3/3
  Demux2/3 -> Switch2/3
  Demux2/2 -> Switch1/3
  Demux2/1 -> Switch/3
  Demux/4 -> Switch3/1
  Demux/3 -> Switch2/1
  Demux/2 -> Switch1/1
  Demux/1 -> Switch/1
  Signal False x4/1 -> Demux2/1
  Signal True x4/1 -> Demux/1
  True/False x4/1 -> Demux1/1
  Mux/1 -> Selected x4/1

== system playback_data/Control/Actuator Control with Torque SEA commands/Timers ==
  Start [1/0] x4 : Inport
  Time [s] : Inport  Port=2
  Demux : Demux
  Mux : Mux
  Sum{8..11} (4 alike) : Sum  Inputs=|-+
  Time on Contact : Subsystem
  Time on Contact1 : Subsystem
  Time on Contact2 : Subsystem
  Time on Contact3 : Subsystem
  Timer [s] x4 : Outport
  wires:
  Sum10/1 -> Mux/3
  Sum11/1 -> Mux/4
  Demux/1 -> Time on Contact/Trigger
  Demux/4 -> Time on Contact3/Trigger
  Demux/3 -> Time on Contact2/Trigger
  Time on Contact3/1(out) -> Sum11/1
  Sum9/1 -> Mux/2
  Start [1/0] x4/1 -> Demux/1
  Sum8/1 -> Mux/1
  Time on Contact1/1(out) -> Sum9/1
  Demux/2 -> Time on Contact1/Trigger
  Time [s]/1 -> Time on Contact3/1(in), Time on Contact2/1(in), Time on Contact1/1(in), Time on Contact/1(in), Sum8/2, Sum9/2, Sum11/2, Sum10/2
  Mux/1 -> Timer [s] x4/1
  Time on Contact2/1(out) -> Sum10/1
  Time on Contact/1(out) -> Sum8/1

== system playback_data/Control/Behavior Control/At Least One Stance Detected ==
  Enable : EnablePort  StatesWhenEnabling=reset
  Constant : Constant
  Stance? : Outport  InitialOutput=[0]
  wires:
  Constant/1 -> Stance?/1

== system playback_data/Control/Behavior Control/Compute Forces1 ==
  XYZ Acceleration : Inport
  Constant5 : Constant  Value=g
  Demux : Demux  Outputs=3
  Gain4 : Gain  Gain=m_total_real
  Mux : Mux  Inputs=3
  Sum8 : Sum  Inputs=|++
  XYZ Force : Outport
  wires:
  Demux/1 -> Mux/1
  Demux/2 -> Mux/2
  Demux/3 -> Sum8/1
  Sum8/1 -> Mux/3
  Mux/1 -> Gain4/1
  Gain4/1 -> XYZ Force/1
  XYZ Acceleration/1 -> Demux/1
  Constant5/1 -> Sum8/2

== system playback_data/Control/Behavior Control/Contact State Machine ==
  Contact Factor [body weight] : Inport
  "[Z dZ] [m m/s]" : Inport  Port=2
  ddZ [m/s^2] : Inport  Port=3
  Contact Factor ddz : Scope
      settings: YMin=-8  YMax=11  SaveName=ScopeData47  SampleInput=on
  Contact State : Scope
      settings: YMin=-0.007  YMax=0.0005  SaveName=ScopeData46  SampleInput=on
  Detect Fall Nonpositive : simulink/Logic and Bit Operations/Detect Fall Nonpositive  vinit=1  InputProcessing=Inherited  OutDataTypeStr=boolean
  Mux : Mux  Inputs=2
  Mux25 : Mux  Inputs=5
  Selector : Selector  InputPortWidth=2  Indices=[2]
  State Machine : State Transition Table  TreatAsAtomicUnit=on
  Unit Delay5 : UnitDelay  SampleTime=-1
  Unit Delay6 : UnitDelay  SampleTime=sample_time
  Unit Delay7 : UnitDelay  InitialCondition=1  SampleTime=sample_time
  flight [1/0] : Outport
  Exiting Stance [1/0] : Outport  Port=2
  wires:
  Detect Fall Nonpositive/1 -> Exiting Stance [1/0]/1
  Unit Delay7/1 -> flight [1/0]/1
  Unit Delay6/1 -> Detect Fall Nonpositive/1
  State Machine/4(" Takeoff") -> Unit Delay6/1, Mux25/4
  Selector/1 -> State Machine/1(z_velocity), Unit Delay5/1
  Contact Factor [body weight]/1 -> Mux/1, State Machine/3(vertical_grf)
  Unit Delay5/1 -> State Machine/2(previous_z_velocity)
  State Machine/5(" Flight") -> Mux25/5, Unit Delay7/1
  Mux25/1 -> Contact State/1
  State Machine/3(" Unloading") -> Mux25/3
  State Machine/2(" LockedContact") -> Mux25/2
  State Machine/1(" TouchDown") -> Mux25/1
  "[Z dZ] [m m/s]"/1 -> Selector/1
  ddZ [m/s^2]/1 -> Mux/2, State Machine/4(vertical_acceleration)
  Mux/1 -> Contact Factor ddz/1

== system playback_data/Control/Behavior Control/Estimate Angular Accelerations2 ==
  Angular Velocities [rad/s] x3 : Inport
  Enabled : Inport  Port=2
  Detect Change : simulink/Logic and Bit Operations/Detect Change  vinit=0  InputProcessing=Inherited  OutDataTypeStr=boolean
  Difference : simulink/Discrete/Difference  ICPrevInput=0.0  InputProcessing=Inherited  OutMin=[]  OutMax=[]  OutDataType=fixdt(1, 16)  OutScaling=2^-10  DoSatur=off
  Gain : Gain  Gain=1/sample_time
  IMU Two Pole Filter1 : DiscreteTransferFcn  Numerator=[A_lpf_imu 0 0]  Denominator=[1 B1_lpf_imu B2_lpf_imu]  SampleTime=sample_time
  Logical Operator5 : Logic  Operator=NOT  AllPortsSameDT=off  OutDataTypeStr=boolean
  Product : Product
  Angular Accelerations [rad/s^2] x3 : Outport
  wires:
  Enabled/1 -> Detect Change/1
  Logical Operator5/1 -> Product/2
  Product/1 -> IMU Two Pole Filter1/1
  Angular Velocities [rad/s] x3/1 -> Difference/1
  Gain/1 -> Product/1
  Difference/1 -> Gain/1
  Detect Change/1 -> Logical Operator5/1
  IMU Two Pole Filter1/1 -> Angular Accelerations [rad/s^2] x3/1

== system playback_data/Control/Behavior Control/Estimate Angular Accelerations3 ==
  Angular Velocities [rad/s] x2 : Inport
  Enabled : Inport  Port=2
  Detect Change : simulink/Logic and Bit Operations/Detect Change  vinit=0  InputProcessing=Inherited  OutDataTypeStr=boolean
  Difference : simulink/Discrete/Difference  ICPrevInput=0.0  InputProcessing=Inherited  OutMin=[]  OutMax=[]  OutDataType=fixdt(1, 16)  OutScaling=2^-10  DoSatur=off
  Gain : Gain  Gain=1/sample_time
  Lateral Angle Two Pole Filter1 : DiscreteTransferFcn  Numerator=[A_lpf_lateral_angle 0 0]  Denominator=[1 B1_lpf_lateral_angle B2_lpf_lateral_angle]  SampleTime=sample_time
  Logical Operator5 : Logic  Operator=NOT  AllPortsSameDT=off  OutDataTypeStr=boolean
  Product : Product
  Angular Accelerations [rad/s^2] x2 : Outport
  wires:
  Detect Change/1 -> Logical Operator5/1
  Difference/1 -> Gain/1
  Gain/1 -> Product/1
  Angular Velocities [rad/s] x2/1 -> Difference/1
  Product/1 -> Lateral Angle Two Pole Filter1/1
  Logical Operator5/1 -> Product/2
  Enabled/1 -> Detect Change/1
  Lateral Angle Two Pole Filter1/1 -> Angular Accelerations [rad/s^2] x2/1

== system playback_data/Control/Behavior Control/Exited Stance ==
  Enable : EnablePort  StatesWhenEnabling=reset
  Constant : Constant
  Takeoff? : Outport  InitialOutput=[0]
  wires:
  Constant/1 -> Takeoff?/1

== system playback_data/Control/Behavior Control/Force Estimation ==
  Right/Left Primary : Inport
  Flight [1/0] : Inport  Port=2
  q : Inport  Port=3
  Torso Roll [rad rad/s] : Inport  Port=4
  Torso Pitch [rad rad/s] : Inport  Port=5
  Torso Yaw [rad rad/s] : Inport  Port=6
  Primary Leg Length [m m/s] : Inport  Port=7
  Primary Leg Angle [rad rad/s] : Inport  Port=8
  Primary Leg Roll [rad rad/s] : Inport  Port=9
  Secondary Leg Roll [rad rad/s] : Inport  Port=10
  Leg Width Right/Left [m m] : Inport  Port=11
  Leg Length Right/Left [m m] : Inport  Port=12
  Primary Lateral Torque [Nm] : Inport  Port=13
  Secondary Lateral Torque [Nm] : Inport  Port=14
  3D Forward Dynamics yawed : MATLAB Function  TreatAsAtomicUnit=on
  Constant : Constant  Value=m_total_real*g
  Demux : Demux  Outputs=2
  Divide : Product  Inputs=*/
  Lateral Motor Saturation : Saturate  UpperLimit=HIP_MTR_MAX_TORQUE  LowerLimit=-HIP_MTR_MAX_TORQUE
      settings: AttributesFormatString=Top: %<UpperLimit>\nBottom: %<LowerLimit>
  Lateral Motor Saturation1 : Saturate  UpperLimit=HIP_MTR_MAX_TORQUE  LowerLimit=-HIP_MTR_MAX_TORQUE
      settings: AttributesFormatString=Top: %<UpperLimit>\nBottom: %<LowerLimit>
  Leg Force Measurements : Subsystem
  Leg Plane GRF : Subsystem
  Logical Operator : Logic  Operator=NOT  AllPortsSameDT=off  OutDataTypeStr=boolean
  Mux : Mux  Inputs=2
  Mux1 : Mux  Inputs=2
  Product : Product
  Product2 : Product
  Product3 : Product
  Selector1 : Selector  InputPortWidth=2  Indices=[1]
  Selector2 : Selector  InputPortWidth=2  Indices=[1]
  Sum : Sum  Inputs=+|+
  Switch1 : Switch  Criteria=u2 ~= 0
  Switch2 : Switch  Criteria=u2 ~= 0
  Switch3 : Switch  Criteria=u2 ~= 0
  two_pole_filter : DiscreteTransferFcn  Numerator=[(1-2*exp(-fcut_contact*sample_time)+exp(-2*fcut_contact*sample_time)) 0 0]  Denominator=[1 (-2*exp(-fcut_contact*sample_time)) (exp(-2*fcut_contact*sample_time))]  SampleTime=sample_time
  Leg Plane Force for Contact Detection [body weight] : Outport
  Right GRF [X Y Z] [N N N] : Outport  Port=2
  Left GRF [X Y Z] [N N N] : Outport  Port=3
  GRF XYZ estimates [N N N] : Outport  Port=4  OutputWhenDisabled=reset  InitialOutput=[0 0 0 0 0 0]
  Torso Roll Acceleration [rad/s^2] : Outport  Port=5  OutputWhenDisabled=reset  InitialOutput=[0 0 0 0 0 0]
  wires:
  Divide/1 -> Leg Plane Force for Contact Detection [body weight]/1
  Leg Width Right/Left [m m]/1 -> Leg Force Measurements/2(Leg Width Right/Left [m m])
  q/1 -> Leg Force Measurements/1(q)
  two_pole_filter/1 -> Divide/1
  Constant/1 -> Divide/2
  [RightLeft] -> 3D Forward Dynamics yawed/1(right_or_left), Switch2/2, Switch1/2
  Leg Length Right/Left [m m]/1 -> Leg Force Measurements/3(Leg Length Right/Left [m m])
  3D Forward Dynamics yawed/1(R_GRF) -> Product2/2
  3D Forward Dynamics yawed/2(L_GRF) -> Product3/1
  3D Forward Dynamics yawed/3(ddroll) -> Product/1
  Leg Force Measurements/3(Right Leg Axial Force [N]) -> Mux/1, Switch1/1
  Leg Force Measurements/4(Left Leg Axial Force [N]) -> Switch1/3, Mux/2
  Switch1/1 -> 3D Forward Dynamics yawed/10(primary_leg_force)
  [TorsoPitch] -> 3D Forward Dynamics yawed/3(torso_pitch)
  Torso Roll [rad rad/s]/1 -> 3D Forward Dynamics yawed/2(torso_roll)
  Torso Yaw [rad rad/s]/1 -> 3D Forward Dynamics yawed/4(torso_yaw)
  Primary Leg Length [m m/s]/1 -> 3D Forward Dynamics yawed/6(primary_leg_length)
  [LegAngle] -> 3D Forward Dynamics yawed/5(primary_sagittal_leg_angle)
  Flight [1/0]/1 -> Logical Operator/1
  [Stance] -> Product/2
  Product/1 -> Torso Roll Acceleration [rad/s^2]/1
  Switch3/1 -> two_pole_filter/1
  Logical Operator/1 -> [Stance]
  Product3/1 -> Left GRF [X Y Z] [N N N]/1, Sum/2
  Product2/1 -> Right GRF [X Y Z] [N N N]/1, Sum/1
  [Stance] -> Product3/2
  [Stance] -> Product2/1
  Primary Leg Roll [rad rad/s]/1 -> 3D Forward Dynamics yawed/7(primary_leg_roll)
  Secondary Leg Roll [rad rad/s]/1 -> 3D Forward Dynamics yawed/8(secondary_leg_roll)
  Switch2/1 -> 3D Forward Dynamics yawed/9(primary_leg_torque)
  Leg Force Measurements/1(Right Leg Torque [Nm]) -> Switch2/1
  Leg Force Measurements/2(Left Leg Torque [Nm]) -> Switch2/3
  Sum/1 -> GRF XYZ estimates [N N N]/1
  Mux1/1 -> Leg Plane GRF/2(Orthogonal Force [N])
  Mux/1 -> Leg Plane GRF/1(Axial Force [N])
  Leg Force Measurements/5(Right Leg Orthogonal Force [N]) -> Mux1/1
  Leg Force Measurements/6(Left Leg Orthogonal Force [N]) -> Mux1/2
  Right/Left Primary/1 -> [RightLeft]
  [RightLeft] -> Switch3/2
  Leg Plane GRF/1(Vertical Force [N]) -> Demux/1
  Demux/1 -> Switch3/1
  Demux/2 -> Switch3/3
  Primary Leg Angle [rad rad/s]/1 -> [LegAngle]
  Torso Pitch [rad rad/s]/1 -> [TorsoPitch]
  [LegAngle] -> Selector1/1
  Selector1/1 -> Leg Plane GRF/4(Leg Angle [rad])
  [TorsoPitch] -> Selector2/1
  Selector2/1 -> Leg Plane GRF/3(Torso Pitch [rad])
  Primary Lateral Torque [Nm]/1 -> Lateral Motor Saturation/1
  Secondary Lateral Torque [Nm]/1 -> Lateral Motor Saturation1/1
  Lateral Motor Saturation/1 -> 3D Forward Dynamics yawed/11(primary_lateral_torque)
  Lateral Motor Saturation1/1 -> 3D Forward Dynamics yawed/12(secondary_lateral_torque)

== system playback_data/Control/Behavior Control/L Leg Calculator ==
  Front [rad rad/s] : Inport
  Back [rad rad/s] : Inport  Port=2
  Constant : Constant  Value=d_ankle_to_foot-0.01
  Demux1 : Demux  Outputs=2
  Gain1 : Gain  Gain=2*l_seg
  Gain2 : Gain  Gain=l_seg
  Gain3 : Gain  Gain=-1
  Gain4 : Gain  Gain=0.5
  Gain5 : Gain  Gain=0.5
  Gain6 : Gain  Gain=2
  Mux1 : Mux  Inputs=2
  Product : Product  RndMeth=Zero
  Sum : Sum  Inputs=++|
  Sum4 : Sum  Inputs=+|+
  Sum5 : Sum  Inputs=+|-
  Trigonometric Function : Trigonometry  Operator=cos
  Trigonometric Function1 : Trigonometry
  "Leg Length [m m/s] " : Outport
  Leg Angle [rad rad/s] : Outport  Port=2
  Leg Splay [rad rad/s] : Outport  Port=3
  w [m] : Outport  Port=4
  wires:
  Sum/1 -> Mux1/1
  Constant/1 -> Sum/1
  Sum4/1 -> Gain5/1
  Mux1/1 -> "Leg Length [m m/s] "/1
  Sum5/1 -> Demux1/1, Leg Splay [rad rad/s]/1
  Gain2/1 -> Gain6/1, Product/1
  Demux1/1 -> Gain4/1
  Gain3/1 -> Product/2
  Demux1/2 -> Gain3/1
  Back [rad rad/s]/1 -> Sum5/1, Sum4/1
  Front [rad rad/s]/1 -> Sum4/2, Sum5/2
  Product/1 -> Mux1/2
  Trigonometric Function1/1 -> Gain2/1
  Gain1/1 -> Sum/2
  Trigonometric Function/1 -> Gain1/1
  Gain4/1 -> Trigonometric Function/1, Trigonometric Function1/1
  Gain6/1 -> w [m]/1
  Gain5/1 -> Leg Angle [rad rad/s]/1

== system playback_data/Control/Behavior Control/Primary Secondary Leg Swap ==
  note: q Order:
      |
      | backJointR
      | backGearR
      | frontJointR
      | frontGearR
      |
      | backJointL
      | backGearL
      | frontJointL
      | frontGearL
      |
      | latR
      | latL
      |
      | boomRoll
      | boomYaw
      | boomPitch
  Exiting Stance [1/0] : Inport
  R Leg Angle [rad rad/s] : Inport  Port=2
  R Leg Length [m m/s] : Inport  Port=3
  R Leg w [m] : Inport  Port=4
  R Back Joint [rad rad/s] : Inport  Port=5
  R Back Gear [rad rad/s] : Inport  Port=6
  R Front Joint [rad rad/s] : Inport  Port=7
  R Front Gear [rad rad/s] : Inport  Port=8
  L Leg Angle [rad rad/s] : Inport  Port=9
  L Leg Length [m m/s] : Inport  Port=10
  L Leg w [m] : Inport  Port=11
  L Back Joint [rad rad/s] : Inport  Port=12
  L Back Gear [rad rad/s] : Inport  Port=13
  L Front Joint [rad rad/s] : Inport  Port=14
  L Front Gear [rad rad/s] : Inport  Port=15
  Primary Back/Front SEA Torque [Nm Nm] : Inport  Port=16
  Secondary Back/Front SEA Torque [Nm Nm] : Inport  Port=17
  "Right Leg Roll [rad, rad/s]" : Inport  Port=18
  "Left Leg Roll [rad, rad/s]" : Inport  Port=19
  Primary Lateral Torque [Nm] : Inport  Port=20
  Secondary Lateral Torque [Nm] : Inport  Port=21
  Primary Front/Back Velocity [rad/s rad/s] : Inport  Port=22
  Secondary Front/Back Velocity [rad/s rad/s] : Inport  Port=23
  Bus Creator : BusCreator  Inputs=22
  Bus Creator1 : BusCreator  Inputs=22
  Bus Selector : BusSelector  OutputSignals=signal1,signal2,signal3,signal4,signal5,signal6,signal7,signal8,signal9,signal10,signal11,signal12,signal13,signal14,signal15,signal16,signal17,signal18,signal19,signal20,signal21,signal22
  Manual Switch : ManualSwitch
  Right Left Primary : Scope
      settings: YMin=-0.007  YMax=0.0005  SaveName=ScopeData48  SampleInput=on
  Select Leg : Constant  Value=initial_leg_selection  OutDataTypeStr=boolean
  Switch6 : Switch  Criteria=u2 ~= 0  OutDataTypeStr=Inherit: Inherit via back propagation  ZeroCross=off
  ToggleRightLeftLeg : MATLAB Function  TreatAsAtomicUnit=on
      settings: MinAlgLoopOccurrences=on
  Unit Delay : UnitDelay  InitialCondition=initial_leg_selection  SampleTime=sample_time
  Right/Left Primary [1/0] : Outport
  Primary Leg Angle [rad rad/s] : Outport  Port=2
  Primary Leg Length [m m/s] : Outport  Port=3
  Primary Leg w [m] : Outport  Port=4
  Primary Back Joint [rad rad/s] : Outport  Port=5
  Primary Back Gear [rad rad/s] : Outport  Port=6
  Primary Front Joint [rad rad/s] : Outport  Port=7
  Primary Front Gear [rad rad/s] : Outport  Port=8
  Secondary Leg Angle [rad rad/s] : Outport  Port=9
  Secondary Leg Length [rad rad/s] : Outport  Port=10
  Secondary Leg w [m] : Outport  Port=11
  Secondary Back Joint [rad rad/s] : Outport  Port=12
  Secondary Back Gear [rad rad/s] : Outport  Port=13
  Secondary Front Joint [rad rad/s] : Outport  Port=14
  Secondary Front Gear [rad rad/s] : Outport  Port=15
  R Back/Front SEA Torque [Nm Nm] : Outport  Port=16
  L Back/Front SEA Torque [Nm Nm] : Outport  Port=17
  "Primary Leg Roll [rad, rad/s]" : Outport  Port=18
  "Secondary Leg Roll [rad, rad/s]" : Outport  Port=19
  Right Lateral Torque [Nm] : Outport  Port=20
  Left Lateral Torque [Nm] : Outport  Port=21
  Right Front/Back Velocity [rad/s rad/s] : Outport  Port=22
  Left Front/Back Velocity [rad/s rad/s] : Outport  Port=23
  wires:
  Unit Delay/1 -> ToggleRightLeftLeg/2(previous_right_left)
  Exiting Stance [1/0]/1 -> ToggleRightLeftLeg/1(toggle)
  ToggleRightLeftLeg/1(right_left) -> Unit Delay/1, Manual Switch/1
  Manual Switch/1 -> Right Left Primary/1, Right/Left Primary [1/0]/1, Switch6/2
  Select Leg/1 -> Manual Switch/2
  R Leg Angle [rad rad/s]/1 -> Bus Creator1/8, Bus Creator/1
  Bus Creator/1 -> Switch6/1
  Bus Creator1/1 -> Switch6/3
  Switch6/1 -> Bus Selector/1
  R Leg Length [m m/s]/1 -> Bus Creator1/9, Bus Creator/2
  R Leg w [m]/1 -> Bus Creator1/10, Bus Creator/3
  R Back Joint [rad rad/s]/1 -> Bus Creator1/11, Bus Creator/4
  R Front Joint [rad rad/s]/1 -> Bus Creator1/13, Bus Creator/6
  R Front Gear [rad rad/s]/1 -> Bus Creator1/14, Bus Creator/7
  L Leg Angle [rad rad/s]/1 -> Bus Creator/8, Bus Creator1/1
  L Leg Length [m m/s]/1 -> Bus Creator1/2, Bus Creator/9
  L Leg w [m]/1 -> Bus Creator1/3, Bus Creator/10
  L Back Joint [rad rad/s]/1 -> Bus Creator1/4, Bus Creator/11
  L Back Gear [rad rad/s]/1 -> Bus Creator1/5, Bus Creator/12
  L Front Joint [rad rad/s]/1 -> Bus Creator1/6, Bus Creator/13
  L Front Gear [rad rad/s]/1 -> Bus Creator1/7, Bus Creator/14
  Primary Back/Front SEA Torque [Nm Nm]/1 -> Bus Creator1/16, Bus Creator/15
  Secondary Back/Front SEA Torque [Nm Nm]/1 -> Bus Creator1/15, Bus Creator/16
  "Right Leg Roll [rad, rad/s]"/1 -> Bus Creator1/18, Bus Creator/17
  "Left Leg Roll [rad, rad/s]"/1 -> Bus Creator1/17, Bus Creator/18
  Primary Lateral Torque [Nm]/1 -> Bus Creator1/20, Bus Creator/19
  Secondary Lateral Torque [Nm]/1 -> Bus Creator1/19, Bus Creator/20
  R Back Gear [rad rad/s]/1 -> Bus Creator1/12, Bus Creator/5
  Bus Selector/1 -> Primary Leg Angle [rad rad/s]/1  "<signal1>"
  Bus Selector/2 -> Primary Leg Length [m m/s]/1  "<signal2>"
  Bus Selector/3 -> Primary Leg w [m]/1  "<signal3>"
  Bus Selector/4 -> Primary Back Joint [rad rad/s]/1  "<signal4>"
  Bus Selector/5 -> Primary Back Gear [rad rad/s]/1  "<signal5>"
  Bus Selector/6 -> Primary Front Joint [rad rad/s]/1  "<signal6>"
  Bus Selector/7 -> Primary Front Gear [rad rad/s]/1  "<signal7>"
  Bus Selector/8 -> Secondary Leg Angle [rad rad/s]/1  "<signal8>"
  Bus Selector/9 -> Secondary Leg Length [rad rad/s]/1  "<signal9>"
  Bus Selector/10 -> Secondary Leg w [m]/1  "<signal10>"
  Bus Selector/11 -> Secondary Back Joint [rad rad/s]/1  "<signal11>"
  Bus Selector/12 -> Secondary Back Gear [rad rad/s]/1  "<signal12>"
  Bus Selector/13 -> Secondary Front Joint [rad rad/s]/1  "<signal13>"
  Bus Selector/14 -> Secondary Front Gear [rad rad/s]/1  "<signal14>"
  Bus Selector/15 -> R Back/Front SEA Torque [Nm Nm]/1  "<signal15>"
  Bus Selector/16 -> L Back/Front SEA Torque [Nm Nm]/1  "<signal16>"
  Bus Selector/17 -> "Primary Leg Roll [rad, rad/s]"/1  "<signal17>"
  Bus Selector/18 -> "Secondary Leg Roll [rad, rad/s]"/1  "<signal18>"
  Bus Selector/19 -> Right Lateral Torque [Nm]/1  "<signal19>"
  Bus Selector/20 -> Left Lateral Torque [Nm]/1  "<signal20>"
  Primary Front/Back Velocity [rad/s rad/s]/1 -> Bus Creator1/22, Bus Creator/21
  Secondary Front/Back Velocity [rad/s rad/s]/1 -> Bus Creator1/21, Bus Creator/22
  Bus Selector/21 -> Right Front/Back Velocity [rad/s rad/s]/1  "<signal21>"
  Bus Selector/22 -> Left Front/Back Velocity [rad/s rad/s]/1  "<signal22>"
